simulink model "simulink_test"  (R2018b)
settings: Solver=FixedStepAuto  StartTime=timeSpan(1)  StopTime=timeSpan(2)  FixedStep=dt  RelTol=1e-3
values from neighbouring files (symbols this model uses):
  ICs = aircraft_data(4:15)    [Input.m]
undefined symbols (not defined in the file or in its folder): forces, Mg, Moments
libraries: shared6dof x1
settings Model: Creator=Dell  LastModifiedBy=OWNER
settings DataIOCC: ReturnWorkspaceOutputs=on
settings DebuggingCC: SFMachineParentedDataDiag=error

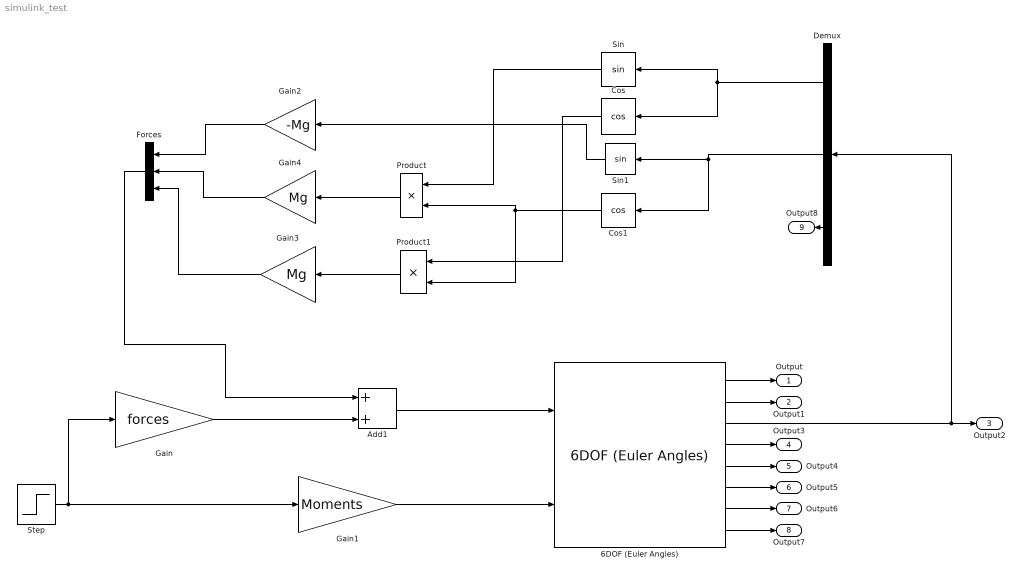
== system simulink_test ==
  6DOF (Euler Angles) : shared6dof/6DOF (Euler Angles)  units=Metric (MKS)  mtype=Fixed  rep=Euler Angles  xme_0=ICs(10:12)  Vm_0=ICs(1:3)  eul_0=ICs(7:9)  pm_0=ICs(4:6)  mass_0=Mass  mass_e=0.5  mass_f=2.0  inertia=I  inertia_e=eye(3)  inertia_f=2*eye(3)  k_quat=1.0  vre_flag=on  abi_flag=off  aMode=0  xme_statename=''  Vm_statename=''  eul_statename=''  quat_statename=''  pm_statename=''  mass_statename=''
      settings: SourceProductBaseCode=AE,PW,DR,MT,UV,VE
  Add1 : Sum
  Cos : Trigonometry  Operator=cos
  Cos1 : Trigonometry  Operator=cos
  Demux : Demux  Outputs=3
  Forces : Concatenate  NumInputs=3
  Gain : Gain  Gain=forces
  Gain1 : Gain  Gain=Moments
  Gain2 : Gain  Gain=-Mg
  Gain3 : Gain  Gain=Mg
  Gain4 : Gain  Gain=Mg
  Product : Product
  Product1 : Product
  Sin : Trigonometry
  Sin1 : Trigonometry
  Step : Step  Time=0  SampleTime=0
  Output : Outport  SignalName=velocities earth  VectorParamsAs1DForOutWhenUnconnected=on
  Output1 : Outport  Port=2  SignalName=positions earth  VectorParamsAs1DForOutWhenUnconnected=on
  Output2 : Outport  Port=3  SignalName=rotational speed earth  VectorParamsAs1DForOutWhenUnconnected=on
  Output3 : Outport  Port=4  VectorParamsAs1DForOutWhenUnconnected=on
  Output4 : Outport  Port=5  SignalName=velocity body  VectorParamsAs1DForOutWhenUnconnected=on
  Output5 : Outport  Port=6  SignalName=rotational speed body  VectorParamsAs1DForOutWhenUnconnected=on
  Output6 : Outport  Port=7  VectorParamsAs1DForOutWhenUnconnected=on
  Output7 : Outport  Port=8  VectorParamsAs1DForOutWhenUnconnected=on
  Output8 : Outport  Port=9  SignalName=don't care  VectorParamsAs1DForOutWhenUnconnected=on
  wires:
  Step/1 -> Gain/1, Gain1/1
  6DOF (Euler Angles)/1 -> Output/1
  6DOF (Euler Angles)/2 -> Output1/1
  6DOF (Euler Angles)/3 -> Demux/1, Output2/1
  6DOF (Euler Angles)/4 -> Output3/1
  6DOF (Euler Angles)/5 -> Output4/1
  6DOF (Euler Angles)/6 -> Output5/1
  6DOF (Euler Angles)/7 -> Output6/1
  6DOF (Euler Angles)/8 -> Output7/1
  Demux/1 -> Sin/1, Cos/1
  Demux/2 -> Cos1/1, Sin1/1
  Gain1/1 -> 6DOF (Euler Angles)/2
  Gain/1 -> Add1/2
  Forces/1 -> Add1/1
  Gain2/1 -> Forces/1
  Gain4/1 -> Forces/2
  Gain3/1 -> Forces/3
  Sin1/1 -> Gain2/1
  Sin/1 -> Product/1
  Cos1/1 -> Product/2, Product1/2
  Product/1 -> Gain4/1
  Cos/1 -> Product1/1
  Product1/1 -> Gain3/1
  Add1/1 -> 6DOF (Euler Angles)/1
  Demux/3 -> Output8/1
